simulink model "SeriesCompTx"  (R2020a)
settings: Solver=VariableStepAuto  StartTime=0.0  StopTime=0.1  RelTol=1e-3
undefined symbols (not defined in the file): D1, Delta
libraries: powerlib x16, powerlib_meascontrol x3
settings Model: Creator=Alisamar  LastModifiedBy=Alisamar

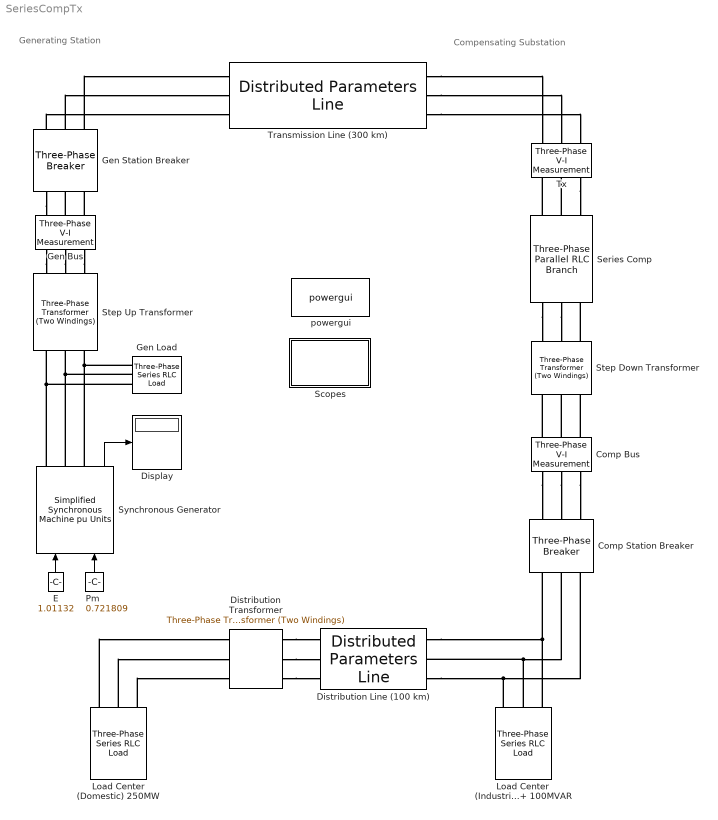
== system SeriesCompTx ==
  note: Compensating Substation
  note: Generating Station
  Comp Bus : powerlib/Measurements/Three-Phase V-I Measurement  VoltageMeasurement=phase-to-ground  SetLabelV=on  LabelV=Comp_Vabc  Vpu=on  VpuLL=off  CurrentMeasurement=yes  SetLabelI=on  LabelI=Comp_Iabc  Ipu=on  Pbase=1000e6  Vbase=230e3  OutputType=Complex  PhasorSimulation=off  PSBequivalent=0
  Comp Station Breaker : powerlib/Elements/Three-Phase Breaker  InitialState=closed  SwitchA=on  SwitchB=on  SwitchC=on  SwitchTimes=[1]  External=off  BreakerResistance=0.01  SnubberResistance=1e5  SnubberCapacitance=0  Measurements=None
  Display : Display
  Distribution Transformer : powerlib/Elements/Three-Phase Transformer (Two Windings)  Winding1Connection=Yg  Winding2Connection=Yg  CoreType=Three single-phase transformers  SetSaturation=off  Hysteresis=off  DataFile='hysteresis'  SetInitialFlux=off  Measurements=None  UNITS=pu  NominalPower=[ 350e6 , 60 ]  Winding1=[ 230e3 , 0.002 , 0.08 ]  Winding2=[ 220 , 0.002 , 0.08 ]  Rm=500  Lm=500  L0=0.5  Saturation=[ 0,0 ; 0.0024,1.2 ; 1.0,1.52 ]  InitialFluxes=[ 0.8 , -0.8 , 0.7 ]  BreakLoop=off  DiscreteSolver=Trapezoidal iterative  DataType=off  TransfoNumber=1
  Distribution Line (100 km) : powerlib/Elements/Distributed Parameters Line  Phases=3  Frequency=60  Resistance=[0.01273 0.3864]  Inductance="[0.9337e-3  4.1264e-3]"  Capacitance=[12.74e-9 7.751e-9]  Length=100  x1=[5.78102978041324e-07 204700.630279113 204700.114604188;376.991118430775 376.991118430775 376.991118430775;0.854207494014601 0.123965458330895 -1.44682650513533]  x2=[4.03373074103655e-07 198814.167762296 198813.666916352;376.991118430775 376.991118430775 376.991118430775;0.313613784935277 -0.0353201032269167 -1.60611206669314]  x3=[1.28425273934898e-09 217.430937936361 217.430390191602;376.991118430775 376.991118430775 376.991118430775;3.11024780143046 2.45768354875485 0.886891585288872]  x4=[2.44049527045548e-09 1660.32316628009 1660.31898364995;376.991118430775 376.991118430775 376.991118430775;0.24320996455731 -0.10042583271949 -1.67121779618567]  x5=0.000565541566995742  V1=[5.781e-07 2.047e+05 2.047e+05;377 377 377;0.8542 0.124 -1.447]  V2=[4.034e-07 1.988e+05 1.988e+05;377 377 377;0.3136 -0.03532 -1.606]  I1=[1.284e-09 217.4 217.4;377 377 377;3.11 2.458 0.8869]  I2=[2.44e-09 1660 1660;377 377 377;0.2432 -0.1004 -1.671]  nHarmo=1  Measurements=None
  E : Constant  Value=1.01132
  Gen Bus : powerlib/Measurements/Three-Phase V-I Measurement  VoltageMeasurement=phase-to-ground  SetLabelV=on  LabelV=Gen_Vabc  Vpu=on  VpuLL=off  CurrentMeasurement=yes  SetLabelI=on  LabelI=Gen_Iabc  Ipu=on  Pbase=1000e6  Vbase=735e3  OutputType=Complex  PhasorSimulation=off  PSBequivalent=0
  Gen Load : powerlib/Elements/Three-Phase Series RLC Load  LConnTagsString=A|B|C  Configuration=Y (grounded)  NominalVoltage=13.8e3  Vabc=[1e3 1e3 1e3]  Vabcp=[1e3 1e3 1e3]  NominalFrequency=60  UnbalancedPower=off  ActivePower=100e3  InductivePower=0  CapacitivePower=0  Pabc=[10e3 9e3 11e3]  QLabc=[100 90 110]  QCabc=[100 90 110]  Pabcp=[10e3 9e3 11e3]  QLabcp=[100 90 110]  QCabcp=[100 90 110]  Measurements=None  LoadType=constant Z
  Gen Station Breaker : powerlib/Elements/Three-Phase Breaker  InitialState=closed  SwitchA=on  SwitchB=on  SwitchC=on  SwitchTimes=[1]  External=off  BreakerResistance=0.01  SnubberResistance=1e5  SnubberCapacitance=0  Measurements=None
  Load Center (Domestic) 250MW : powerlib/Elements/Three-Phase Series RLC Load  LConnTagsString=A|B|C  Configuration=Y (grounded)  NominalVoltage=220  Vabc=[1e3 1e3 1e3]  Vabcp=[1e3 1e3 1e3]  NominalFrequency=60  UnbalancedPower=off  ActivePower=250e6  InductivePower=0  CapacitivePower=0  Pabc=[10e3 9e3 11e3]  QLabc=[100 90 110]  QCabc=[100 90 110]  Pabcp=[10e3 9e3 11e3]  QLabcp=[100 90 110]  QCabcp=[100 90 110]  Measurements=None  LoadType=constant Z
  Load Center (Industrial) 650MW + 100MVAR : powerlib/Elements/Three-Phase Series RLC Load  LConnTagsString=A|B|C  Configuration=Y (grounded)  NominalVoltage=230e3  Vabc=[1e3 1e3 1e3]  Vabcp=[1e3 1e3 1e3]  NominalFrequency=60  UnbalancedPower=off  ActivePower=650e6  InductivePower=100e6  CapacitivePower=0  Pabc=[10e3 9e3 11e3]  QLabc=[100 90 110]  QCabc=[100 90 110]  Pabcp=[10e3 9e3 11e3]  QLabcp=[100 90 110]  QCabcp=[100 90 110]  Measurements=None  LoadType=constant Z
  Pm : Constant  Value=0.721809
  Scopes : Subsystem
  Series Comp : powerlib/Elements/Three-Phase Parallel RLC Branch  LConnTagsString=A|B|C  RConnTagsString=A|B|C  BranchType=C  Resistance=1  Inductance=1e-3  Capacitance=128e-3  Measurements=None
      settings: SourceProductBaseCode=PS
  Step Down Transformer : powerlib/Elements/Three-Phase Transformer (Two Windings)  Winding1Connection=Yg  Winding2Connection=Yg  CoreType=Three single-phase transformers  SetSaturation=off  Hysteresis=off  DataFile='hysteresis'  SetInitialFlux=off  Measurements=None  UNITS=pu  NominalPower=[ 1000e6 , 60 ]  Winding1=[ 735e3 , 0.002 , 0.08 ]  Winding2=[ 230e3 , 0.002 , 0.08 ]  Rm=500  Lm=500  L0=0.5  Saturation=[ 0,0 ; 0.0024,1.2 ; 1.0,1.52 ]  InitialFluxes=[0 0 0]  BreakLoop=off  DiscreteSolver=Trapezoidal iterative  DataType=off  TransfoNumber=1
  Step Up Transformer : powerlib/Elements/Three-Phase Transformer (Two Windings)  Winding1Connection=Delta (D1)  Winding2Connection=Yg  CoreType=Three single-phase transformers  SetSaturation=off  Hysteresis=off  DataFile='hysteresis'  SetInitialFlux=off  Measurements=None  UNITS=pu  NominalPower=[ 1500e6 , 60 ]  Winding1=[ 13.8e3 , 0.002 , 0.08 ]  Winding2=[ 735e3 , 0.002 , 0.08 ]  Rm=500  Lm=500  L0=0.5  Saturation=[ 0,0 ; 0.0024,1.2 ; 1.0,1.52 ]  InitialFluxes=[ 0.8 , -0.8 , 0.7 ]  BreakLoop=off  DiscreteSolver=Trapezoidal iterative  DataType=off  TransfoNumber=1
  Synchronous Generator : powerlib/Machines/Simplified Synchronous Machine pu Units  ConnectionType=3-wire Y  MechanicalLoad=Mechanical power Pm  MeasurementBus=off  NominalParameters="[ 1200e6 13.8e3  60 ]"  Mechanical=[ inf,0,2 ]  InternalRL="[ 0.22/15  0.22 ]"  InitialConditions=[0 1.43122 0.716215 0.716215 0.716215 -3.34575 -123.346 116.654 ]  IterativeDiscreteModel=Trapezoidal non iterative  TsBlock=-1  TsPowergui=0  LoadFlowParameters=[1,0,0,0,0]  Units=0  BusType=PV  Pref=1000000000  Qref=0  Qmin=-Inf  Qmax=Inf  PLF=0  QLF=0
      settings: AttributesFormatString=\n  SourceProductBaseCode=MT,PS
  Transmission Line (300 km) : powerlib/Elements/Distributed Parameters Line  Phases=3  Frequency=60  Resistance=[0.01273 0.3864]  Inductance="[0.9337e-3  4.1264e-3]"  Capacitance=[12.74e-9 7.751e-9]  Length=300  x1=[1.78593719315789e-06 671880.076722127 671878.384145135;376.991118430775 376.991118430775 376.991118430775;-0.43976560275591 0.161443063768676 -1.40934889969753]  x2=[1.5744070204634e-06 677706.082360895 677704.375107206;376.991118430775 376.991118430775 376.991118430775;-1.06345632069096 0.00044461542954595 -1.57034734803656]  x3=[1.69543313573239e-10 1492.33491548882 1492.33115605106;376.991118430775 376.991118430775 376.991118430775;-1.47188549507784 -0.176770834531894 -1.74756279799784]  x4=[3.94763083190861e-09 3523.49554195185 3523.48666568334;376.991118430775 376.991118430775 376.991118430775;-1.04752005077614 -0.0890438687307339 -1.65983583219696]  x5=0.00169662470098723  V1=[1.786e-06 6.719e+05 6.719e+05;377 377 377;-0.4398 0.1614 -1.409]  V2=[1.574e-06 6.777e+05 6.777e+05;377 377 377;-1.063 0.0004446 -1.57]  I1=[1.695e-10 1492 1492;377 377 377;-1.472 -0.1768 -1.748]  I2=[3.948e-09 3523 3523;377 377 377;-1.048 -0.08904 -1.66]  nHarmo=1  Measurements=None
  Tx : powerlib/Measurements/Three-Phase V-I Measurement  VoltageMeasurement=phase-to-ground  SetLabelV=on  LabelV=Tx_Vabc  Vpu=on  VpuLL=off  CurrentMeasurement=yes  SetLabelI=on  LabelI=Tx_Iabc  Ipu=on  Pbase=1000e6  Vbase=735e3  OutputType=Complex  PhasorSimulation=off  PSBequivalent=0
  powergui : powerlib/powergui  Priority=1  SimulationMode=Continuous  SampleTime=50e-6  frequency=60  Iterations=50  frequencyindice=0  Pbase=100e6  ErrMax=1e-4  UnitsV=kV  UnitsW=MW  buscounter=0  FunctionMessages=off  echomessages=off  EnableUseOfTLC=off  CurrentSourceSwitches=off  DisableSnubberDevices=off  DisableRonSwitches=off  DisableVfSwitches=off  DisplayEquations=off  AutomaticDiscreteSolvers=off  SolverType=Tustin/Backward Euler (TBE)  Interpol=off  ExternalGateDelay=off  methode=off  Ts=100  x0status=blocks  SPID=on  SwTol=0  HookPort=off  NonlinearTolerance=1e-4  nMaxIteration=100  ContinueOnMaxIteration=off  RestoreLinks=warning  ResistiveCurrentMeasurement=off  Frange=[0:2:500]  Ylog=off  Xlog=on  ShowGrid=off  save=off  variable=ZData  structure=0  ZoomFFT=off  StartTime=0.0  cycles=1  DisplayStyle=1  fundamental=60  FreqAxis=off  MaxFrequency=1000  frequencyindicesteady=1  RmsSteady=1  display=off
  wires:
  Synchronous Generator/1 -> Display/1
  Pm/1 -> Synchronous Generator/1
  E/1 -> Synchronous Generator/2
  connections:
  Load Center (Domestic) 250MW/LConn1 -- Distribution Transformer/RConn1
  Load Center (Domestic) 250MW/LConn2 -- Distribution Transformer/RConn2
  Load Center (Domestic) 250MW/LConn3 -- Distribution Transformer/RConn3
  Distribution Transformer/LConn3 -- Distribution Line (100 km)/RConn3
  Distribution Transformer/LConn2 -- Distribution Line (100 km)/RConn2
  Distribution Transformer/LConn1 -- Distribution Line (100 km)/RConn1
  Gen Station Breaker/RConn2 -- Transmission Line (300 km)/LConn2
  Gen Station Breaker/RConn1 -- Transmission Line (300 km)/LConn1
  Gen Station Breaker/LConn3 -- Gen Bus/RConn3
  Gen Bus/RConn2 -- Gen Station Breaker/LConn2
  Gen Bus/RConn1 -- Gen Station Breaker/LConn1
  Gen Station Breaker/RConn3 -- Transmission Line (300 km)/LConn3
  Gen Bus/LConn1 -- Step Up Transformer/RConn1
  Gen Bus/LConn2 -- Step Up Transformer/RConn2
  Gen Load/LConn3 -- Synchronous Generator/RConn3 -- Step Up Transformer/LConn3
  Gen Load/LConn2 -- Synchronous Generator/RConn2 -- Step Up Transformer/LConn2
  Gen Load/LConn1 -- Synchronous Generator/RConn1 -- Step Up Transformer/LConn1
  Gen Bus/LConn3 -- Step Up Transformer/RConn3
  Load Center (Industrial) 650MW + 100MVAR/LConn2 -- Comp Station Breaker/RConn2 -- Distribution Line (100 km)/LConn2
  Load Center (Industrial) 650MW + 100MVAR/LConn3 -- Distribution Line (100 km)/LConn1 -- Comp Station Breaker/RConn1
  Load Center (Industrial) 650MW + 100MVAR/LConn1 -- Distribution Line (100 km)/LConn3 -- Comp Station Breaker/RConn3
  Tx/RConn3 -- Series Comp/LConn3
  Series Comp/LConn2 -- Tx/RConn2
  Series Comp/LConn1 -- Tx/RConn1
  Transmission Line (300 km)/RConn3 -- Tx/LConn3
  Transmission Line (300 km)/RConn2 -- Tx/LConn2
  Transmission Line (300 km)/RConn1 -- Tx/LConn1
  Comp Bus/LConn3 -- Step Down Transformer/RConn3
  Comp Bus/LConn2 -- Step Down Transformer/RConn2
  Comp Bus/LConn1 -- Step Down Transformer/RConn1
  Comp Bus/RConn1 -- Comp Station Breaker/LConn1
  Comp Bus/RConn2 -- Comp Station Breaker/LConn2
  Comp Bus/RConn3 -- Comp Station Breaker/LConn3
  Step Down Transformer/LConn3 -- Series Comp/RConn3
  Series Comp/RConn2 -- Step Down Transformer/LConn2
  Series Comp/RConn1 -- Step Down Transformer/LConn1

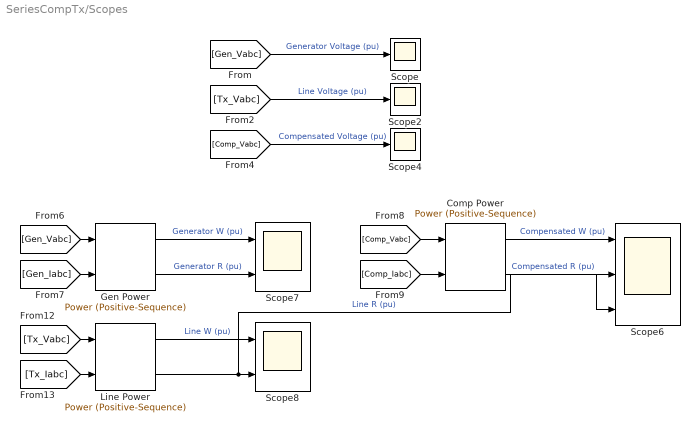
== system SeriesCompTx/Scopes ==
  Comp Power : powerlib_meascontrol/Measurements/Power (Positive-Sequence)  Freq=60  Vinit=[0, 0]  Iinit=[0, 0]  Ts=0
      settings: SourceProductBaseCode=PS
  Gen Power : powerlib_meascontrol/Measurements/Power (Positive-Sequence)  Freq=60  Vinit=[0, 0]  Iinit=[0, 0]  Ts=0
      settings: SourceProductBaseCode=PS
  Line Power : powerlib_meascontrol/Measurements/Power (Positive-Sequence)  Freq=60  Vinit=[0, 0]  Iinit=[0, 0]  Ts=0
      settings: SourceProductBaseCode=PS
  Scope : Scope
  Scope2 : Scope
  Scope4 : Scope
  Scope6 : Scope  NumInputPorts=3
  Scope7 : Scope  NumInputPorts=2
  Scope8 : Scope  NumInputPorts=2
  wires:
  [Gen_Vabc] -> Scope/1  "Generator Voltage (pu)"
  [Tx_Vabc] -> Scope2/1  "Line Voltage (pu)"
  [Comp_Vabc] -> Scope4/1  "Compensated Voltage (pu)"
  [Gen_Vabc] -> Gen Power/1
  [Gen_Iabc] -> Gen Power/2
  Gen Power/1 -> Scope7/1  "Generator W (pu)"
  Gen Power/2 -> Scope7/2  "Generator R (pu)"
  Comp Power/2 -> Scope6/3  "Compensated R (pu)"
  Comp Power/1 -> Scope6/1  "Compensated W (pu)"
  [Comp_Iabc] -> Comp Power/2
  [Comp_Vabc] -> Comp Power/1
  [Tx_Vabc] -> Line Power/1
  [Tx_Iabc] -> Line Power/2
  Line Power/1 -> Scope8/1  "Line W (pu)"
  Line Power/2 -> Scope6/2, Scope8/2  "Line R (pu)"
